simulink model "UnitDelayConqatTo6"  (Simulink 7.6)
settings: Solver=ode45  StartTime=0.0  StopTime=10.0  RelTol=1e-3
settings Model: Creator=DominikC  LastModifiedBy=DominikC
settings DebuggingCC: FcnCallInpInsideContextMsg=Enable All

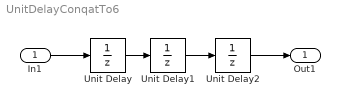
== system UnitDelayConqatTo6 ==
  In1 : Inport
  Unit Delay : UnitDelay  SampleTime=2
  Unit Delay1 : UnitDelay  SampleTime=-1
  Unit Delay2 : UnitDelay  SampleTime=3
  Out1 : Outport
  wires:
  In1/1 -> Unit Delay/1
  Unit Delay/1 -> Unit Delay1/1
  Unit Delay1/1 -> Unit Delay2/1
  Unit Delay2/1 -> Out1/1
